simulink model "main"  (R2016b)
settings: Solver=VariableStepAuto  StartTime=0.0  StopTime=30  FixedStep=Par.Step_size  RelTol=1e-3
values from neighbouring files (symbols this model uses):
  eta_0 = [0 0 0]    [init.m]
  K_psi = 0.28    [init.m]
  nu_0 = [0 0 0]    [init.m]
undefined symbols (not defined in the file or in its folder): now, Par
settings Model: Creator=Ørjan  LastModifiedBy=Ørjan
settings RTWCC: RTWCompilerOptimization=on
settings CodeAppCC: MaxIdLength=95

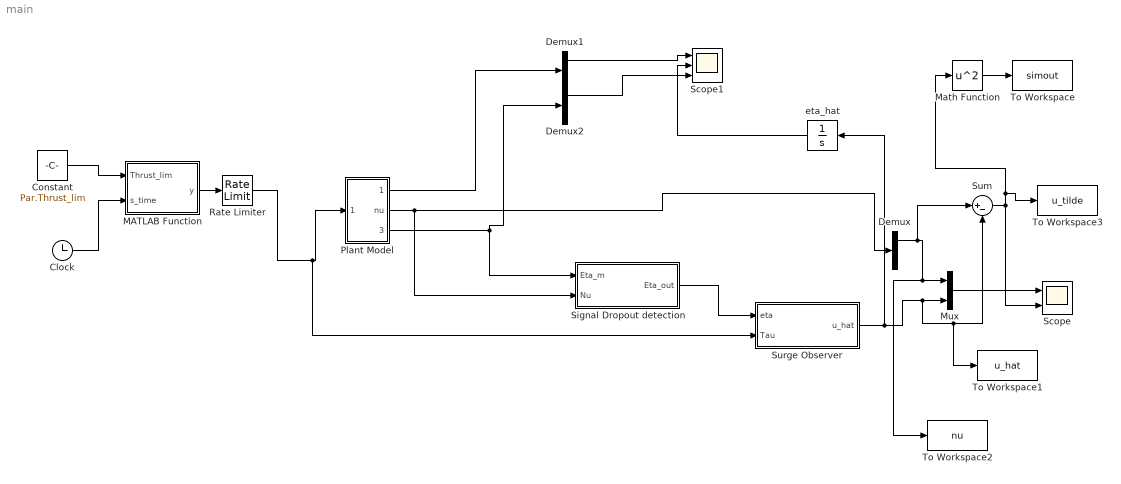
== system main ==
  Clock : Clock
  Constant : Constant  Value=Par.Thrust_lim
  Demux : Demux  Outputs=3
  Demux1 : Demux  Outputs=3
  Demux2 : Demux  Outputs=3
  MATLAB Function : MATLAB Function  TreatAsAtomicUnit=on
  Math Function : Math  Operator=square  SaturateOnIntegerOverflow=on
  Mux : Mux  Inputs=2
  Plant Model : Subsystem
  Rate Limiter : RateLimiter  RisingSlewLimit=5  FallingSlewLimit=-5  SampleTimeMode=inherited
  Scope : Scope  NumInputPorts=2
  Scope1 : Scope  NumInputPorts=3
  Signal Dropout detection : Subsystem
  Sum : Sum  Inputs=|+-
  Surge Observer : Subsystem
  To Workspace : ToWorkspace  VariableName=simout  SaveFormat=Timeseries  SampleTime=-1
  To Workspace1 : ToWorkspace  VariableName=u_hat  SaveFormat=Timeseries  SampleTime=-1
  To Workspace2 : ToWorkspace  VariableName=nu  SaveFormat=Timeseries  SampleTime=-1
  To Workspace3 : ToWorkspace  VariableName=u_tilde  SaveFormat=Timeseries  SampleTime=-1
  eta_hat : Integrator
  wires:
  Surge Observer/1(u_hat) -> eta_hat/1, To Workspace1/1, Sum/2, Mux/2
  Mux/1 -> Scope/1
  Plant Model/2(nu) -> Signal Dropout detection/2(Nu), Demux/1
  Demux/1 -> Sum/1, Mux/1, To Workspace2/1
  Plant Model/3(eta_m) -> Demux2/1, Signal Dropout detection/1(Eta_m)
  Sum/1 -> To Workspace3/1, Math Function/1, Scope/2
  Plant Model/1(eta) -> Demux1/1
  Demux1/1 -> Scope1/1
  eta_hat/1 -> Scope1/2
  Math Function/1 -> To Workspace/1
  Constant/1 -> MATLAB Function/1(Thrust_lim)
  Clock/1 -> MATLAB Function/2(s_time)
  Demux2/1 -> Scope1/3
  Signal Dropout detection/1(Eta_out) -> Surge Observer/1(eta)
  MATLAB Function/1(y) -> Rate Limiter/1
  Rate Limiter/1 -> Surge Observer/2(Tau), Plant Model/1(tau)

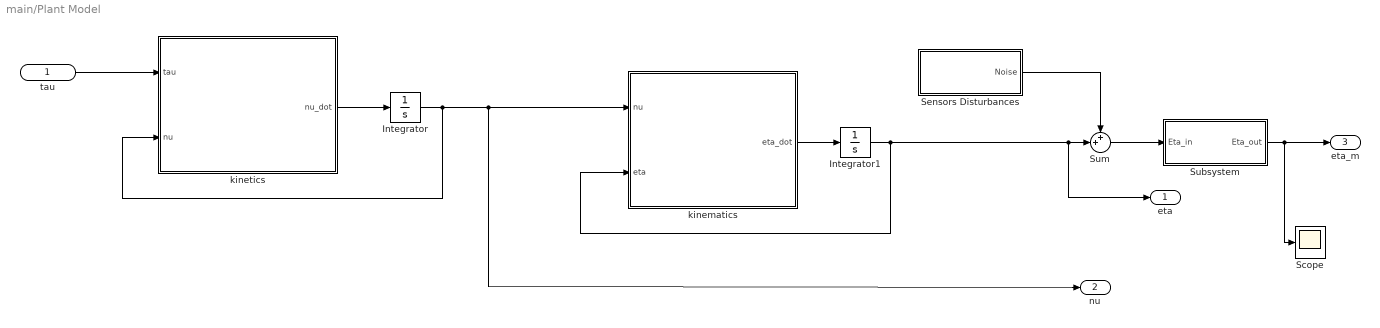
== system main/Plant Model ==
  tau : Inport
  Integrator : Integrator  InitialCondition=nu_0
  Integrator1 : Integrator  InitialCondition=eta_0
  Scope : Scope
  Sensors Disturbances : Subsystem
  Subsystem : Subsystem
  Sum : Sum  Inputs=++|
  kinematics : MATLAB Function  TreatAsAtomicUnit=on
  kinetics : MATLAB Function  TreatAsAtomicUnit=on
  eta : Outport
  nu : Outport  Port=2
  eta_m : Outport  Port=3
  wires:
  tau/1 -> kinetics/1(tau)
  kinetics/1(nu_dot) -> Integrator/1
  kinematics/1(eta_dot) -> Integrator1/1
  Integrator/1 -> kinetics/2(nu), nu/1, kinematics/1(nu)
  Integrator1/1 -> eta/1, Sum/2, kinematics/2(eta)
  Sensors Disturbances/1(Noise) -> Sum/1
  Subsystem/1(Eta_out) -> Scope/1, eta_m/1
  Sum/1 -> Subsystem/1(Eta_in)

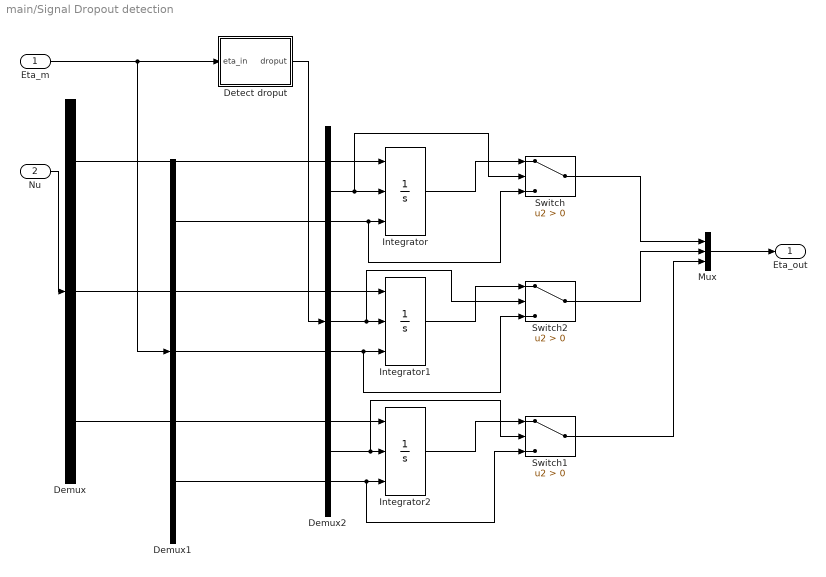
== system main/Signal Dropout detection ==
  Eta_m : Inport
  Nu : Inport  Port=2
  Demux : Demux  Outputs=3
  Demux1 : Demux  Outputs=3
  Demux2 : Demux  Outputs=3
  Detect droput : MATLAB Function  TreatAsAtomicUnit=on
  Integrator : Integrator  ExternalReset=rising  InitialConditionSource=external
  Integrator1 : Integrator  ExternalReset=rising  InitialConditionSource=external
  Integrator2 : Integrator  ExternalReset=rising  InitialConditionSource=external
  Mux : Mux  Inputs=3
  Switch : Switch  Criteria=u2 > Threshold
  Switch1 : Switch  Criteria=u2 > Threshold
  Switch2 : Switch  Criteria=u2 > Threshold
  Eta_out : Outport
  wires:
  Nu/1 -> Demux/1
  Eta_m/1 -> Detect droput/1(eta_in), Demux1/1
  Detect droput/1(droput) -> Demux2/1
  Switch/1 -> Mux/1
  Switch2/1 -> Mux/2
  Switch1/1 -> Mux/3
  Mux/1 -> Eta_out/1
  Demux/1 -> Integrator/1
  Demux/3 -> Integrator2/1
  Demux/2 -> Integrator1/1
  Demux1/1 -> Switch/3, Integrator/3
  Demux1/3 -> Switch1/3, Integrator2/3
  Demux1/2 -> Switch2/3, Integrator1/3
  Demux2/1 -> Switch/2, Integrator/2
  Demux2/3 -> Switch1/2, Integrator2/2
  Demux2/2 -> Switch2/2, Integrator1/2
  Integrator/1 -> Switch/1
  Integrator1/1 -> Switch2/1
  Integrator2/1 -> Switch1/1

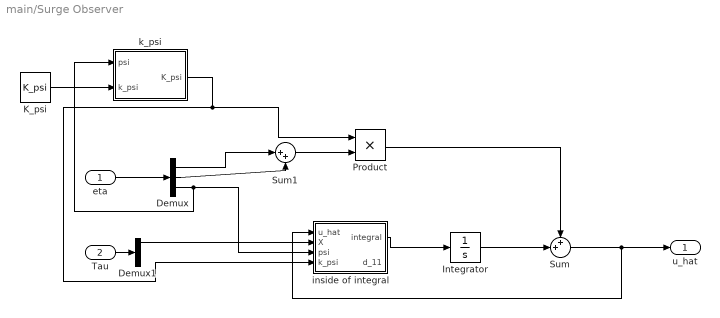
== system main/Surge Observer ==
  eta : Inport
  Tau : Inport  Port=2
  Demux : Demux  Outputs=3
  Demux1 : Demux  Outputs=3
  Integrator : Integrator
  K_psi : Constant  Value=K_psi
  Product : Product
  Sum : Sum  Inputs=++|
  Sum1 : Sum  Inputs=|++
  inside of integral : MATLAB Function  TreatAsAtomicUnit=on
  k_psi : MATLAB Function  TreatAsAtomicUnit=on
  u_hat : Outport
  wires:
  eta/1 -> Demux/1
  inside of integral/1(integral) -> Integrator/1
  Demux/1 -> Sum1/1
  Sum1/1 -> Product/2
  k_psi/1(K_psi) -> inside of integral/4(k_psi), Product/1
  Product/1 -> Sum/1
  Integrator/1 -> Sum/2
  Tau/1 -> Demux1/1
  Demux1/1 -> inside of integral/2(X)
  Demux/3 -> k_psi/1(psi), inside of integral/3(psi)
  Sum/1 -> inside of integral/1(u_hat), u_hat/1
  K_psi/1 -> k_psi/2(k_psi)
  Demux/2 -> Sum1/2

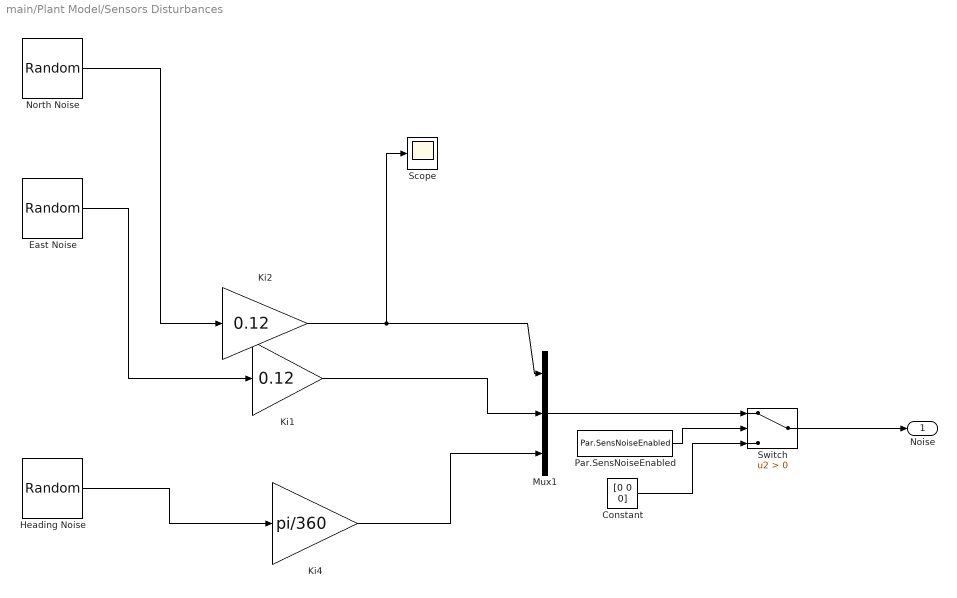
== system main/Plant Model/Sensors Disturbances ==
  Constant : Constant  Value=[0 0 0]
  East Noise : RandomNumber  DisableCoverage=on  Seed=ceil(abs(5*round(abs(now*1e6 - fix(now*1e6))*1e5)))  SampleTime=Par.Sample_time  VectorParams1D=off
  Heading Noise : RandomNumber  DisableCoverage=on  Seed=ceil(abs(11*round(abs(now*1e6 - fix(now*1e6))*1e5)))  SampleTime=Par.Sample_time
  Ki1 : Gain  Gain=0.12  RndMeth=Nearest
  Ki2 : Gain  Gain=0.12  RndMeth=Nearest
  Ki4 : Gain  Gain=pi/360  RndMeth=Nearest
  Mux1 : Mux  Inputs=3
  North Noise : RandomNumber  DisableCoverage=on  Seed=ceil(abs(3*round(abs(now*1e6 - fix(now*1e6))*1e5)))  SampleTime=Par.Sample_time
  Par.SensNoiseEnabled : Constant  Value=Par.SensNoiseEnabled
  Scope : Scope
  Switch : Switch  Criteria=u2 > Threshold
  Noise : Outport
  wires:
  Ki1/1 -> Mux1/2
  Ki2/1 -> Scope/1, Mux1/1
  Par.SensNoiseEnabled/1 -> Switch/2
  Switch/1 -> Noise/1
  Constant/1 -> Switch/3
  Mux1/1 -> Switch/1
  North Noise/1 -> Ki2/1
  East Noise/1 -> Ki1/1
  Heading Noise/1 -> Ki4/1
  Ki4/1 -> Mux1/3

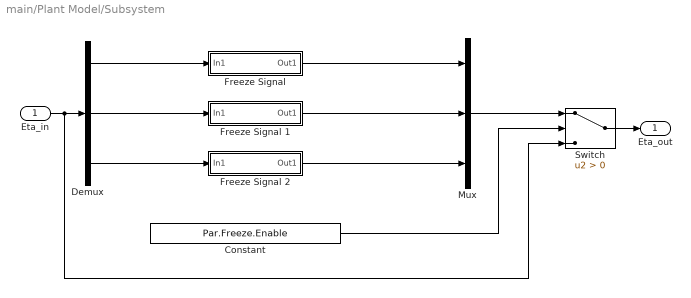
== system main/Plant Model/Subsystem ==
  Eta_in : Inport
  Constant : Constant  Value=Par.Freeze.Enable
  Demux : Demux  Outputs=3
  "Freeze Signal " : Subsystem
  Freeze Signal 1 : Subsystem
  Freeze Signal 2 : Subsystem
  Mux : Mux  Inputs=3
  Switch : Switch  Criteria=u2 > Threshold
  Eta_out : Outport
  wires:
  Eta_in/1 -> Switch/3, Demux/1
  Mux/1 -> Switch/1
  Demux/1 -> "Freeze Signal "/1(In1)
  "Freeze Signal "/1(Out1) -> Mux/1
  Freeze Signal 1/1(Out1) -> Mux/2
  Demux/2 -> Freeze Signal 1/1(In1)
  Demux/3 -> Freeze Signal 2/1(In1)
  Freeze Signal 2/1(Out1) -> Mux/3
  Constant/1 -> Switch/2
  Switch/1 -> Eta_out/1

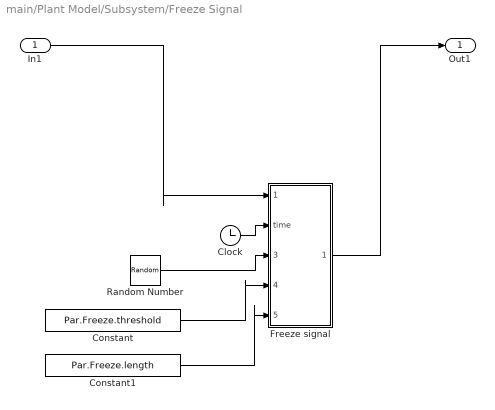
== system main/Plant Model/Subsystem/Freeze Signal  ==
  In1 : Inport
  Clock : Clock
  Constant : Constant  Value=Par.Freeze.threshold
  Constant1 : Constant  Value=Par.Freeze.length
  Freeze signal : MATLAB Function  TreatAsAtomicUnit=on
  Random Number : RandomNumber  Seed=ceil(abs(5*round(abs(now*1e6 - fix(now*1e6))*1e5)))  SampleTime=0.1
  Out1 : Outport
  wires:
  Constant1/1 -> Freeze signal/5(length)
  In1/1 -> Freeze signal/1(eta_in)
  Freeze signal/1(eta_out) -> Out1/1
  Constant/1 -> Freeze signal/4(threshold)
  Clock/1 -> Freeze signal/2(time)
  Random Number/1 -> Freeze signal/3(random_value)

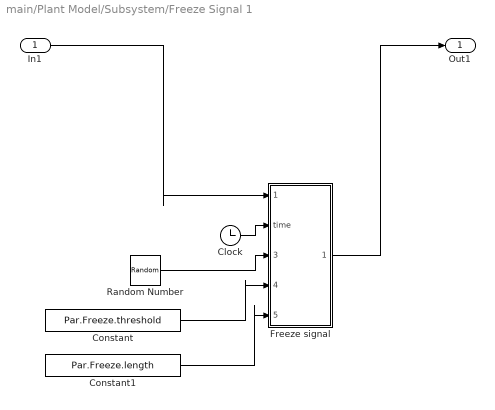
== system main/Plant Model/Subsystem/Freeze Signal 1 ==
  In1 : Inport
  Clock : Clock
  Constant : Constant  Value=Par.Freeze.threshold
  Constant1 : Constant  Value=Par.Freeze.length
  Freeze signal : MATLAB Function  TreatAsAtomicUnit=on
  Random Number : RandomNumber  Seed=ceil(abs(5*round(abs(now*1e6 - fix(now*1e6))*1e5)))  SampleTime=0.1
  Out1 : Outport
  wires:
  Constant1/1 -> Freeze signal/5(length)
  In1/1 -> Freeze signal/1(eta_in)
  Freeze signal/1(eta_out) -> Out1/1
  Constant/1 -> Freeze signal/4(threshold)
  Clock/1 -> Freeze signal/2(time)
  Random Number/1 -> Freeze signal/3(random_value)

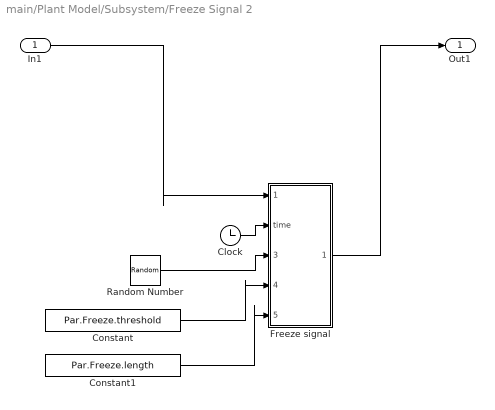
== system main/Plant Model/Subsystem/Freeze Signal 2 ==
  In1 : Inport
  Clock : Clock
  Constant : Constant  Value=Par.Freeze.threshold
  Constant1 : Constant  Value=Par.Freeze.length
  Freeze signal : MATLAB Function  TreatAsAtomicUnit=on
  Random Number : RandomNumber  Seed=ceil(abs(5*round(abs(now*1e6 - fix(now*1e6))*1e5)))  SampleTime=0.1
  Out1 : Outport
  wires:
  Constant1/1 -> Freeze signal/5(length)
  In1/1 -> Freeze signal/1(eta_in)
  Freeze signal/1(eta_out) -> Out1/1
  Constant/1 -> Freeze signal/4(threshold)
  Clock/1 -> Freeze signal/2(time)
  Random Number/1 -> Freeze signal/3(random_value)

== matlab function main/Plant Model/kinematics ==
  data: nu input; eta_dot output; eta input
function eta_dot = CSE1_eta_dot(nu,eta)

psi = eta(3);

J = [cos(psi) -sin(psi) 0
     sin(psi) cos(psi)  0
     0        0         1];

eta_dot = J*nu;

== matlab function main/Plant Model/kinetics ==
  data: tau input; nu_dot output; nu input
function nu_dot = CSE1_nu_dot(tau,nu)

u   = nu(1);
v   = nu(2);
r   = nu(3);

tau = [tau(1);tau(2);tau(3)];
%% MATRICES

m    = 14.79;   I_z  =  1.7600;   x_g = 0.0375;       % x_g  =  0.0460; % Table B.1


%% Added mass
X_ud  =     -2.0;											% Table B.1
					Y_vd =     -1.0;	N_vd =    -0.0;		% Table B.1 guestimate
					Y_rd =      -0.0;	N_rd =    -1.0;		% Table B.1

%% Total mass matrix
m_11 = m-X_ud;
m_22 = m-Y_vd;
m_23 = m*x_g-Y_rd;
m_32 = m*x_g-N_vd;
m_33 = I_z-N_rd;

M    = [m_11 0    0
        0    m_22 m_23
        0    m_32 m_33];
	
%% Damping coefficients
% Comments at the end of the lines indicate the old values used.
X_u		= -0.6555;		X_v		= 0;
X_uu 	= 0.3545;		X_vv	= -2.443;
X_uuu 	= -3.787;		X_vvv	= 0;

						Y_v		= -1.33; 			Y_r		= -7.250; % Y_r
						Y_vv	= -2.776;			Y_rr	= -3.450; % Y_rr
						Y_vvv	= -64.91;			Y_rrr	= 0;
						
						Y_rv	= -0.805;			Y_vr	= -0.845; % Y_rv, Y_vr

						N_v		= 0;				N_r		= -1.900; % N_r
						N_vv	= -0.2088;			N_rr	= -0.750; % N_rr
						N_vvv	= 0;				N_rrr	= 0;
						
						N_rv	= 0.130;			N_vr	= 0.080; % N_rv, N_vr

%% Correolis matrix
c_13 = -(m-Y_vd)*v-(m*x_g-Y_rd)*r;
c_23 = (m-X_ud)*u;
C    = [0     0     c_13
        0     0     c_23
        -c_13 -c_23 0   ];

%% Assembly of the damping matrix
d_11 = -X_u - X_uu*u - X_uuu*u^2;
d_22 = -Y_v - Y_vv*v - Y_vvv*v^2 - Y_rv*abs(r);
d_33 = -N_r - N_rr*abs(r) - N_rrr*r^2 - N_vr*abs(v); % using abs(r)

d_12 = -X_v - X_vv*v - X_vvv*v^2;
d_23 = -Y_r - Y_rr*abs(r) - Y_rrr*r^2 - Y_vr*abs(v);
d_32 = -N_v - N_vv*v - N_vvv*v^2 - N_rv*abs(r);

D    = [d_11 d_12 0
        0    d_22 d_23
        0    d_32 d_33];



%% CALCULATION
nu_dot = M\(tau-(C+D)*nu);

== matlab function main/Surge Observer/inside of integral ==
  data: u_hat input; integral output; X input; psi input; k_psi input; d_11 output
function [integral,d_11] = fcn(u_hat, X, psi, k_psi)
%#codegen
X_u = -.6555;
X_uu = .3545;
X_uuu = -3.787;
m_11 = 16.79;
d_11 = -X_u -X_uu*abs(u_hat) - X_uuu*u_hat^2;
integral = -d_11*u_hat/m_11 + X/m_11 - k_psi*(cos(psi) + sin(psi))*u_hat;
end

== matlab function main/MATLAB Function ==
  data: y output; Thrust_lim input; s_time input
function y = fcn(Thrust_lim, s_time)
coder.extrinsic('get_param');
    y = [0 0 0]';
    if (s_time < 2)
        y_t = [1 0 0];
    elseif (s_time < 4)
        y_t = [1 0 0];
    elseif (s_time <6)
        y_t = [0.5 0 0];
    elseif s_time <8
        y_t = [0 0 0];
    else
        y_t = [0 0 0];
    end
    y = y_t'.*Thrust_lim;
end

== matlab function main/Surge Observer/k_psi ==
  data: psi input; k_psi input; K_psi output
function K_psi = fcn(psi,k_psi)
%#codegen
K_psi = k_psi*sign(sin(psi) + cos(psi));
% y = u;

== matlab function main/Signal Dropout detection/Detect droput ==
  data: eta_in input; droput output
function droput = fcn(eta_in)
persistent eta_old;
if isempty(eta_old)
    eta_old = eta_in;
end
droput = (eta_in - eta_old) == 0;
eta_old = eta_in;
end

== matlab function main/Plant Model/Subsystem/Freeze Signal /Freeze signal ==
  data: eta_in input; eta_out output; time input; random_value input; threshold input; length input
function eta_out = fcn(eta_in, time, random_value, threshold, length)
persistent eta t_1;
if isempty(eta)
    eta = eta_in;
    t_1 = 0;
end

if random_value > threshold
    t_1 = time + length*(0.5*rand+0.5);
end
if time>=t_1
    eta = eta_in;
end

eta_out = eta;
end

== matlab function main/Plant Model/Subsystem/Freeze Signal 1/Freeze signal ==
  data: eta_in input; eta_out output; time input; random_value input; threshold input; length input
function eta_out = fcn(eta_in, time, random_value, threshold, length)
persistent eta t_1;
if isempty(eta)
    eta = eta_in;
    t_1 = 0;
end

if random_value > threshold
    t_1 = time + length*(0.5*rand+0.5);
end
if time>=t_1
    eta = eta_in;
end

eta_out = eta;
end

== matlab function main/Plant Model/Subsystem/Freeze Signal 2/Freeze signal ==
  data: eta_in input; eta_out output; time input; random_value input; threshold input; length input
function eta_out = fcn(eta_in, time, random_value, threshold, length)
persistent eta t_1;
if isempty(eta)
    eta = eta_in;
    t_1 = 0;
end

if random_value > threshold
    t_1 = time + length*(0.5*rand+0.5);
end
if time>=t_1
    eta = eta_in;
end

eta_out = eta;
end
